simulink model "Ex_Feb_2014_5"  (R2022b)
settings: Solver=VariableStepAuto  StartTime=0.0  StopTime=150  RelTol=1e-3
settings Model: Creator=rrilo  LastModifiedBy=rrilo

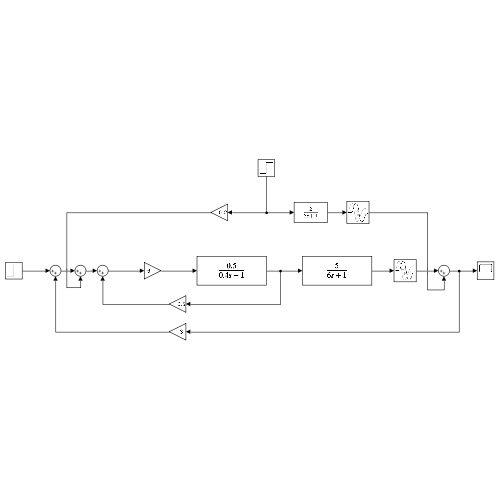
[thumbnail: Simulink's stored preview of the top-level diagram]
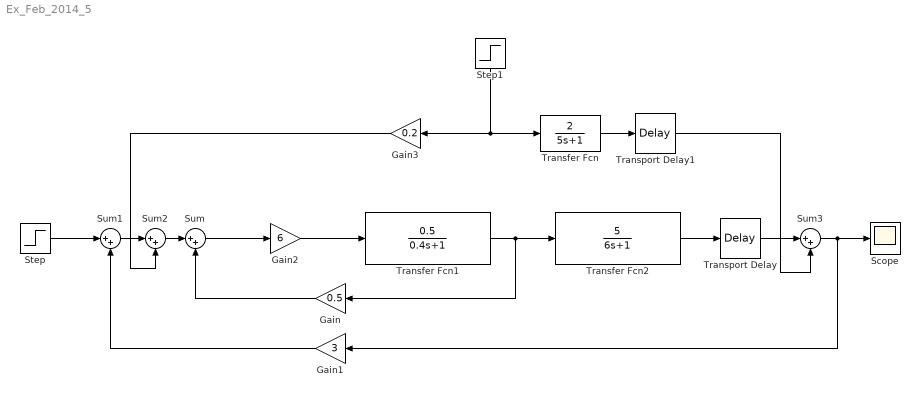
== system Ex_Feb_2014_5 ==
  Gain : Gain  Gain=0.5
  Gain1 : Gain  Gain=3
  Gain2 : Gain  Gain=6
  Gain3 : Gain  Gain=0.2
  Scope : Scope
  Step : Step  SampleTime=0
  Step1 : Step  SampleTime=0
  Sum{,1..3} (4 alike) : Sum  Inputs=|++
  Transfer Fcn : TransferFcn  Numerator=[2]  Denominator=[5 1]
  Transfer Fcn1 : TransferFcn  Numerator=[0.5]  Denominator=[0.4 1]
  Transfer Fcn2 : TransferFcn  Numerator=[5]  Denominator=[6 1]
  Transport Delay : TransportDelay  DelayTime=2
  Transport Delay1 : TransportDelay  DelayTime=6
  wires:
  Gain1/1 -> Sum1/2
  Step/1 -> Sum1/1
  Gain/1 -> Sum/2
  Transfer Fcn2/1 -> Transport Delay/1
  Transfer Fcn1/1 -> Gain/1, Transfer Fcn2/1
  Gain2/1 -> Transfer Fcn1/1
  Sum/1 -> Gain2/1
  Transfer Fcn/1 -> Transport Delay1/1
  Step1/1 -> Gain3/1, Transfer Fcn/1
  Gain3/1 -> Sum2/2
  Sum1/1 -> Sum2/1
  Sum2/1 -> Sum/1
  Transport Delay/1 -> Sum3/1
  Transport Delay1/1 -> Sum3/2
  Sum3/1 -> Gain1/1, Scope/1
